simulink model "Modelo_No_lineal_LeyDeControlM"  (R2023b)
settings: Solver=VariableStepAuto  StartTime=0.0  StopTime=10.0  RelTol=1e-3
values from neighbouring files (symbols this model uses):
  alpha_cu = 3.9e-3    (= 0.0039)    [parametros_proyecto2.m]
  g = 9.81    [parametros_proyecto2.m]
  lambda_m = 0.016    [parametros_proyecto2.m]
  Ld = 6.6e-3    (= 0.0066)    [parametros_proyecto2.m]
  Lq = 5.8e-3    (= 0.0058)    [parametros_proyecto2.m]
  r = 120    [parametros_proyecto2.m]
  Rs_ref = 1.02    [parametros_proyecto2.m]
  Rts_amb = 146.7    [parametros_proyecto2.m]
  Ts0 = 25    [parametros_proyecto2.m]
undefined symbols (not defined in the file or in its folder): b_eq, cts, J_eq, k_l, L_d, L_ls, L_q, magnitude, P_p
settings Model: Creator=ignab  LastModifiedBy=MSI

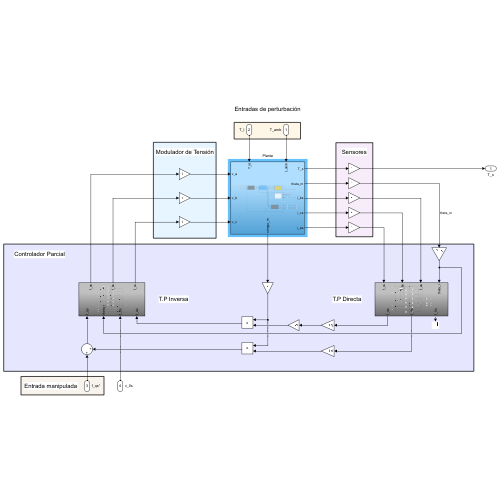
[thumbnail: Simulink's stored preview of the top-level diagram]
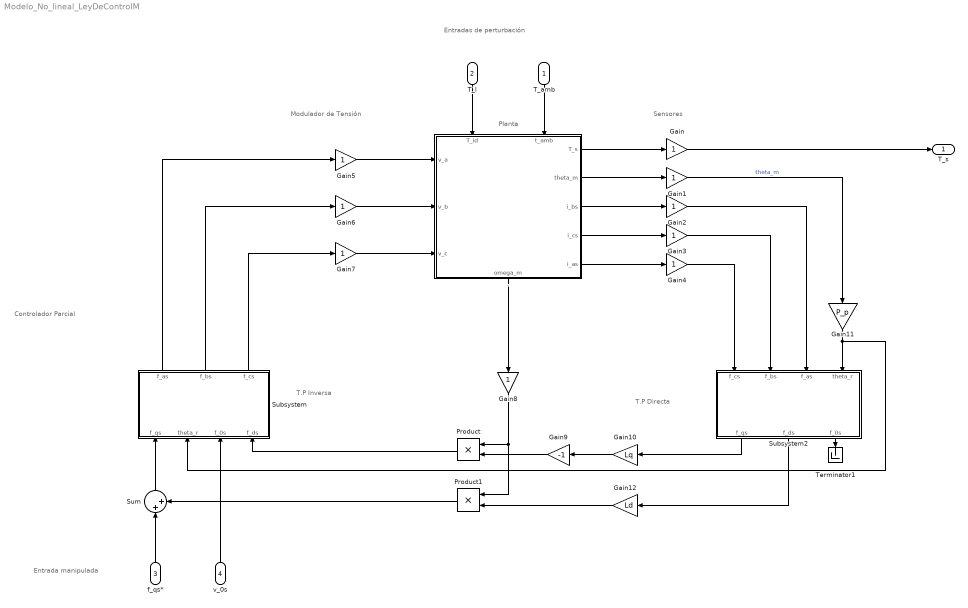
== system Modelo_No_lineal_LeyDeControlM ==
  note: Planta
  note: Modulador de Tensión
  note: Sensores
  note: Entradas de perturbación
  note: Controlador Parcial
  note: T.P Inversa
  note: T.P Directa
  note: Entrada manipulada
  T_amb : Inport
  T_l : Inport  Port=2
  f_qs* : Inport  Port=3
  v_0s : Inport  Port=4
  . : Subsystem
      settings: PortSchema="{\"entries\":[{\"content\":{\"sides\":[{\"content\":{\"connectorIds\":[\"In1\",\"In2\",\"In3\"]},\"type\":\"ConnectorPlacement.EquallySpacedRectSide\",\"uuid\":\"a2221977-a2db-4f9f-a6b6-e4e93ab83132\"},{\"content\":{\"connectorIds\":[\"Out1\",\"Out2\",\"Out3\",\"Out4\",\"Out5\"],\"side\":\"RIGHT\"},\"type\":\"ConnectorPlacement.EquallySpacedRectSide\",\"uuid\":\"4d1b64fb-cd5f-444c-9c55-dd968f667727\"},{\"content\":{\"connectorIds\":[\"In4\",\"In5\"],\"side\":\"TOP\"},\"type\":\"ConnectorPlacement.EquallySpacedRectSide\",\"uuid\":\"feec2d7e-2013-4827-9d2d-5413e6a364ce\"},{\"content\":{\"connectorIds\":[\"Out6\"],\"side\":\"BOTTOM\"},\"type\":\"ConnectorPlacement.EquallySpacedRectSide\",\"uuid\":\"a4e68a75-7272-4a37-88ea-97e0fe693470\"}]},\"type\":\"ConnectorPlacement.EquallySpacedConnector\",\"uuid\":\"3fef7616-1be8-4199-84fe-e5c97ae42ef2\"}],\"packageUris\":[\"http://schema.mathworks.com/mf0/Connector/R2020b\"],\"version\":\"1.0\"}"
  Gain{,1..8} (9 alike) : Gain
  Gain10 : Gain  Gain=Lq
  Gain11 : Gain  Gain=P_p
  Gain12 : Gain  Gain=Ld
  Gain9 : Gain  Gain=-1
  Product : Product
  Product1 : Product
  Subsystem : Subsystem
  Subsystem2 : Subsystem
  Sum : Sum  Inputs=|++
  Terminator1 : Terminator
  T_s : Outport
  wires:
  Subsystem/1(f_as) -> Gain5/1
  Gain5/1 -> ./1(v_a)
  Subsystem/2(f_bs) -> Gain6/1
  Gain6/1 -> ./2(v_b)
  Subsystem/3(f_cs) -> Gain7/1
  Gain7/1 -> ./3(v_c)
  v_0s/1 -> Subsystem/3(f_0s)
  T_l/1 -> ./4(T_id)
  T_amb/1 -> ./5(t_amb)
  ./3(i_bs) -> Gain2/1
  ./4(i_cs) -> Gain3/1
  ./1(T_s) -> Gain/1
  ./2(theta_m) -> Gain1/1
  ./5(i_as) -> Gain4/1
  ./6(omega_m) -> Gain8/1
  Gain/1 -> T_s/1
  Gain1/1 -> Gain11/1  "theta_m"
  Gain11/1 -> Subsystem/2(theta_r), Subsystem2/4(theta_r)
  Gain2/1 -> Subsystem2/3(f_as)
  Gain3/1 -> Subsystem2/2(f_bs)
  Gain4/1 -> Subsystem2/1(f_cs)
  Gain8/1 -> Product1/1, Product/1
  Subsystem2/1(f_qs) -> Gain10/1
  Gain10/1 -> Gain9/1
  Gain9/1 -> Product/2
  Product/1 -> Subsystem/4(f_ds)
  Subsystem2/2(f_ds) -> Gain12/1
  Subsystem2/3(f_0s) -> Terminator1/1
  Gain12/1 -> Product1/2
  f_qs*/1 -> Sum/1
  Sum/1 -> Subsystem/1(f_qs)
  Product1/1 -> Sum/2

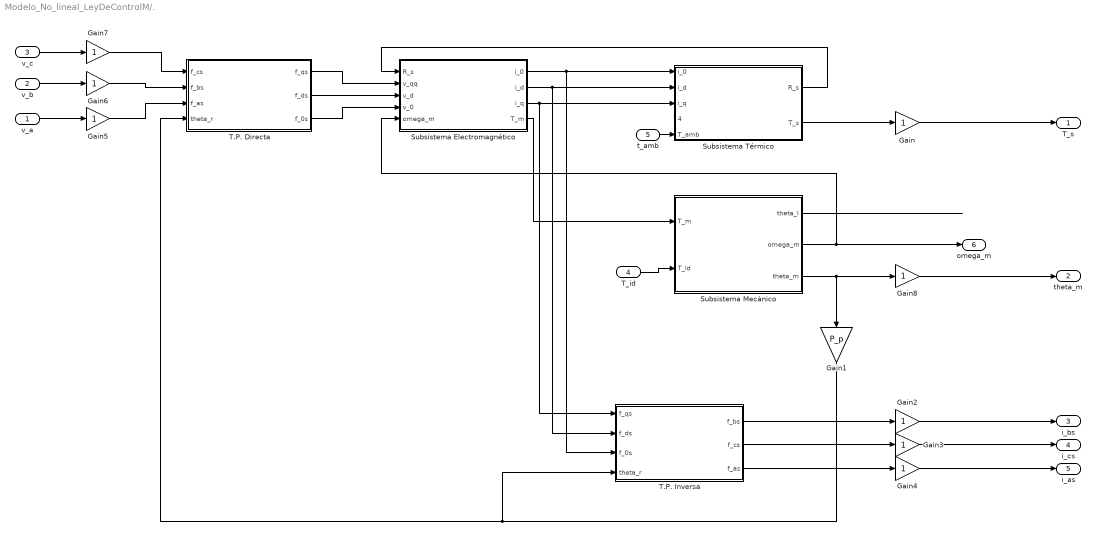
== system Modelo_No_lineal_LeyDeControlM/. ==
  v_a : Inport
  v_b : Inport  Port=2
  v_c : Inport  Port=3
  T_id : Inport  Port=4
  t_amb : Inport  Port=5
  Gain{,2..8} (8 alike) : Gain
  Gain1 : Gain  Gain=P_p
  Subsistema Electromagnético : Subsystem
  Subsistema Mecánico : Subsystem
  Subsistema Térmico : Subsystem
  T.P. Directa : Subsystem
  T.P. Inversa : Subsystem
  T_s : Outport
  theta_m : Outport  Port=2
  i_bs : Outport  Port=3
  i_cs : Outport  Port=4
  i_as : Outport  Port=5
  omega_m : Outport  Port=6
  wires:
  Subsistema Térmico/1(R_s) -> Subsistema Electromagnético/1(R_s)
  T.P. Directa/1(f_qs) -> Subsistema Electromagnético/2(v_qq)
  T.P. Inversa/1(f_bs) -> Gain2/1
  Subsistema Mecánico/2(omega_m) -> Subsistema Electromagnético/5(omega_m), omega_m/1
  Subsistema Electromagnético/1(i_0) -> Subsistema Térmico/1(i_0), T.P. Inversa/3(f_0s)
  Subsistema Mecánico/3(theta_m) -> Gain1/1, Gain8/1
  Gain6/1 -> T.P. Directa/2(f_bs)
  Subsistema Electromagnético/4(T_m) -> Subsistema Mecánico/1(T_m)
  Gain3/1 -> i_cs/1
  Subsistema Mecánico/1(theta_l) -> ?
  Subsistema Electromagnético/2(i_d) -> T.P. Inversa/2(f_ds), Subsistema Térmico/2(i_d)
  Gain2/1 -> i_bs/1
  t_amb/1 -> Subsistema Térmico/5(T_amb)
  v_b/1 -> Gain6/1
  v_c/1 -> Gain7/1
  v_a/1 -> Gain5/1
  Subsistema Térmico/2(T_s) -> Gain/1
  Subsistema Electromagnético/3(i_q) -> T.P. Inversa/1(f_qs), Subsistema Térmico/3(i_q)
  Gain4/1 -> i_as/1
  T.P. Inversa/3(f_as) -> Gain4/1
  T.P. Directa/3(f_0s) -> Subsistema Electromagnético/4(v_0)
  T_id/1 -> Subsistema Mecánico/2(T_ld)
  T.P. Inversa/2(f_cs) -> Gain3/1
  Gain8/1 -> theta_m/1
  Gain7/1 -> T.P. Directa/1(f_cs)
  Gain/1 -> T_s/1
  Gain1/1 -> T.P. Directa/4(theta_r), T.P. Inversa/4(theta_r)
  T.P. Directa/2(f_ds) -> Subsistema Electromagnético/3(v_d)
  Gain5/1 -> T.P. Directa/3(f_as)

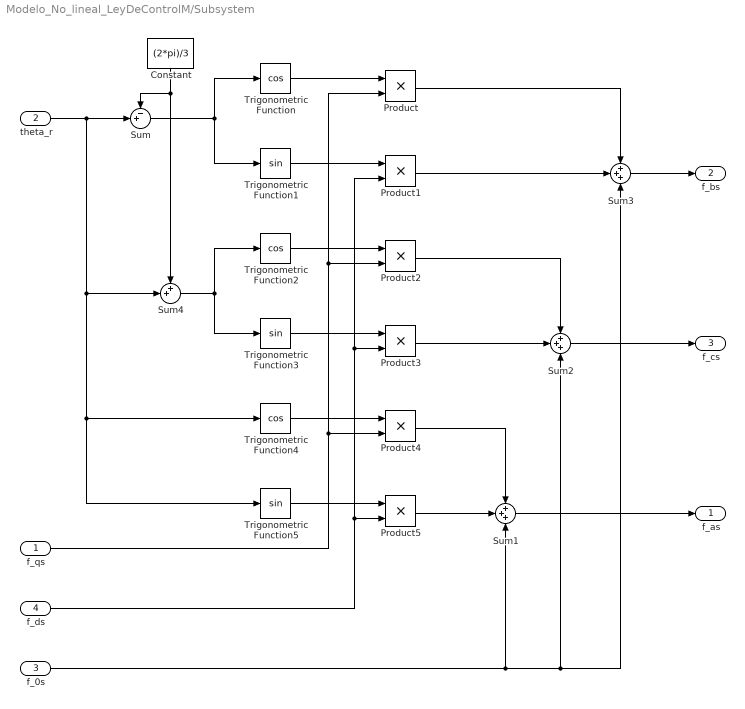
== system Modelo_No_lineal_LeyDeControlM/Subsystem ==
  f_qs : Inport
  theta_r : Inport  Port=2
  f_0s : Inport  Port=3
  f_ds : Inport  Port=4
  Constant : Constant  Value=(2*pi)/3
  Product{,1..5} (6 alike) : Product
  Sum : Sum  Inputs=-+|
  Sum1 : Sum  Inputs=+++
  Sum2 : Sum  Inputs=+++
  Sum3 : Sum  Inputs=+++
  Sum4 : Sum  Inputs=++|
  Trigonometric Function : Trigonometry  Operator=cos
  Trigonometric Function1 : Trigonometry
  Trigonometric Function2 : Trigonometry  Operator=cos
  Trigonometric Function3 : Trigonometry
  Trigonometric Function4 : Trigonometry  Operator=cos
  Trigonometric Function5 : Trigonometry
  f_as : Outport
  f_bs : Outport  Port=2
  f_cs : Outport  Port=3
  wires:
  Sum1/1 -> f_as/1
  Product5/1 -> Sum1/2
  Sum2/1 -> f_cs/1
  Product1/1 -> Sum3/2
  Trigonometric Function5/1 -> Product5/1
  Sum/1 -> Trigonometric Function1/1, Trigonometric Function/1
  Product2/1 -> Sum2/1
  Product4/1 -> Sum1/1
  f_qs/1 -> Product4/2, Product2/2, Product/2
  Product/1 -> Sum3/1
  f_0s/1 -> Sum3/3, Sum2/3, Sum1/3
  Trigonometric Function4/1 -> Product4/1
  Constant/1 -> Sum4/1, Sum/1
  Trigonometric Function2/1 -> Product2/1
  f_ds/1 -> Product5/2, Product3/2, Product1/2
  Trigonometric Function3/1 -> Product3/1
  Trigonometric Function1/1 -> Product1/1
  Sum4/1 -> Trigonometric Function3/1, Trigonometric Function2/1
  Sum3/1 -> f_bs/1
  theta_r/1 -> Sum4/2, Trigonometric Function5/1, Trigonometric Function4/1, Sum/2
  Product3/1 -> Sum2/2
  Trigonometric Function/1 -> Product/1

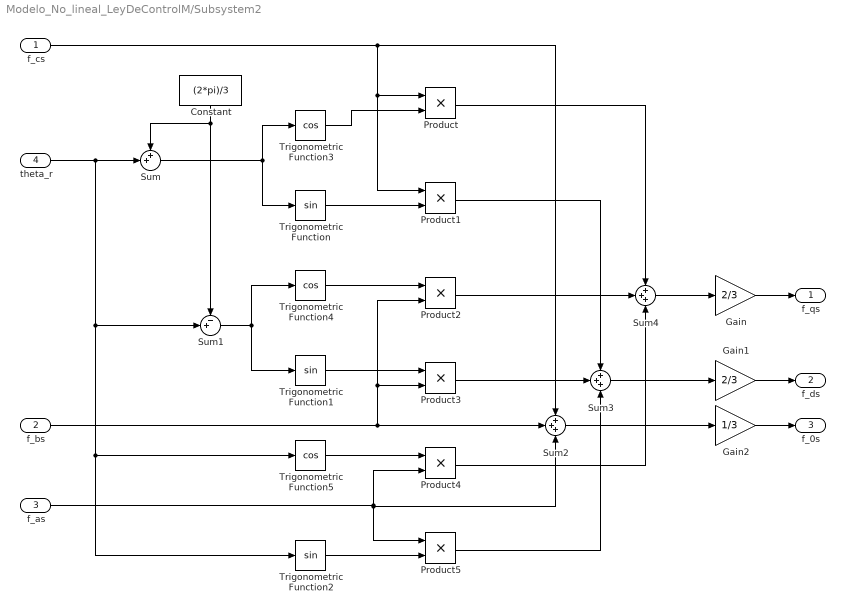
== system Modelo_No_lineal_LeyDeControlM/Subsystem2 ==
  f_cs : Inport
  f_bs : Inport  Port=2
  f_as : Inport  Port=3
  theta_r : Inport  Port=4
  Constant : Constant  Value=(2*pi)/3
  Gain : Gain  Gain=2/3
  Gain1 : Gain  Gain=2/3
  Gain2 : Gain  Gain=1/3
  Product{,1..5} (6 alike) : Product
  Sum : Sum  Inputs=++|
  Sum1 : Sum  Inputs=-+|
  Sum2 : Sum  Inputs=+++
  Sum3 : Sum  Inputs=+++
  Sum4 : Sum  Inputs=+++
  Trigonometric Function : Trigonometry
  Trigonometric Function1 : Trigonometry
  Trigonometric Function2 : Trigonometry
  Trigonometric Function3 : Trigonometry  Operator=cos
  Trigonometric Function4 : Trigonometry  Operator=cos
  Trigonometric Function5 : Trigonometry  Operator=cos
  f_qs : Outport
  f_ds : Outport  Port=2
  f_0s : Outport  Port=3
  wires:
  f_cs/1 -> Product/1, Product1/1, Sum2/1
  Product3/1 -> Sum3/2
  Trigonometric Function5/1 -> Product4/1
  Constant/1 -> Sum/1, Sum1/1
  Sum1/1 -> Trigonometric Function1/1, Trigonometric Function4/1
  Gain2/1 -> f_0s/1
  Gain1/1 -> f_ds/1
  theta_r/1 -> Sum1/2, Trigonometric Function2/1, Trigonometric Function5/1, Sum/2
  Sum4/1 -> Gain/1
  Trigonometric Function1/1 -> Product3/1
  f_bs/1 -> Product2/2, Product3/2, Sum2/2
  Product4/1 -> Sum4/3
  Gain/1 -> f_qs/1
  Product/1 -> Sum4/1
  f_as/1 -> Sum2/3, Product5/1, Product4/2
  Sum2/1 -> Gain2/1
  Product2/1 -> Sum4/2
  Trigonometric Function2/1 -> Product5/2
  Sum3/1 -> Gain1/1
  Trigonometric Function/1 -> Product1/2
  Trigonometric Function3/1 -> Product/2
  Trigonometric Function4/1 -> Product2/1
  Product5/1 -> Sum3/3
  Product1/1 -> Sum3/1
  Sum/1 -> Trigonometric Function3/1, Trigonometric Function/1

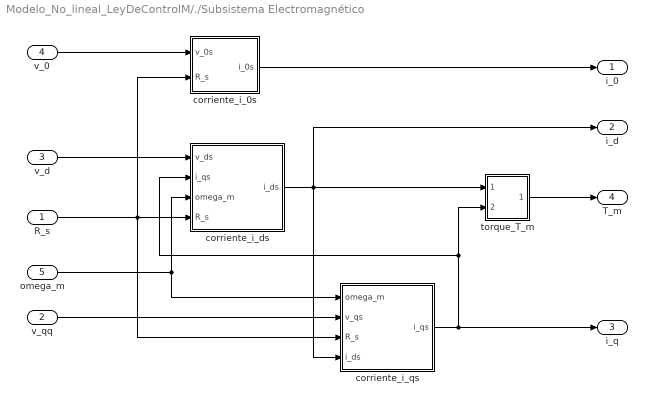
== system Modelo_No_lineal_LeyDeControlM/./Subsistema Electromagnético ==
  R_s : Inport
  v_qq : Inport  Port=2
  v_d : Inport  Port=3
  v_0 : Inport  Port=4
  omega_m : Inport  Port=5
  corriente_i_0s : Subsystem
  corriente_i_ds : Subsystem
  corriente_i_qs : Subsystem
  torque_T_m : Subsystem
  i_0 : Outport
  i_d : Outport  Port=2
  i_q : Outport  Port=3
  T_m : Outport  Port=4
  wires:
  R_s/1 -> corriente_i_qs/3(R_s), corriente_i_ds/4(R_s), corriente_i_0s/2(R_s)
  corriente_i_0s/1(i_0s) -> i_0/1
  corriente_i_qs/1(i_qs) -> i_q/1, torque_T_m/2(i_qs), corriente_i_ds/2(i_qs)
  corriente_i_ds/1(i_ds) -> corriente_i_qs/4(i_ds), torque_T_m/1(i_ds), i_d/1
  v_0/1 -> corriente_i_0s/1(v_0s)
  v_d/1 -> corriente_i_ds/1(v_ds)
  omega_m/1 -> corriente_i_qs/1(omega_m), corriente_i_ds/3(omega_m)
  v_qq/1 -> corriente_i_qs/2(v_qs)
  torque_T_m/1(T_m) -> T_m/1

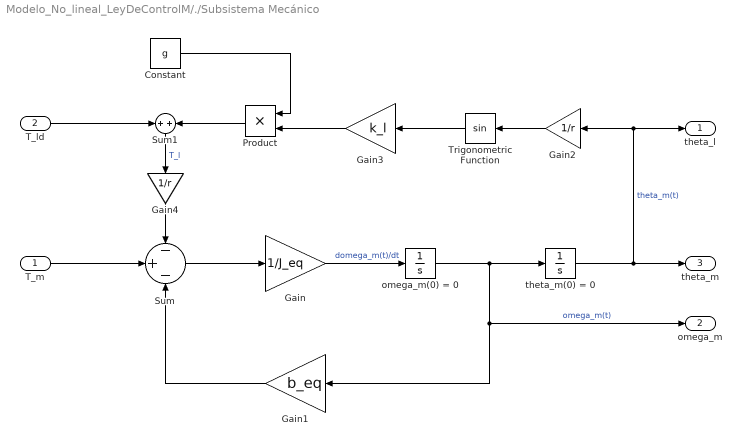
== system Modelo_No_lineal_LeyDeControlM/./Subsistema Mecánico ==
  T_m : Inport
  T_ld : Inport  Port=2
  Constant : Constant  Value=g
  Gain : Gain  Gain=1/J_eq
  Gain1 : Gain  Gain=b_eq
  Gain2 : Gain  Gain=1/r
  Gain3 : Gain  Gain=k_l
  Gain4 : Gain  Gain=1/r
  Product : Product
  Sum : Sum  Inputs=-+-
  Sum1 : Sum
  Trigonometric Function : Trigonometry
  "omega_m(0) = 0\t" : Integrator
  theta_m(0) = 0 : Integrator
  theta_l : Outport
  omega_m : Outport  Port=2
  theta_m : Outport  Port=3
  wires:
  Product/1 -> Sum1/2
  Constant/1 -> Product/1
  T_m/1 -> Sum/2
  Gain3/1 -> Product/2
  T_ld/1 -> Sum1/1
  Gain1/1 -> Sum/3
  Gain4/1 -> Sum/1
  Sum1/1 -> Gain4/1  "T_l"
  theta_m(0) = 0/1 -> theta_l/1, Gain2/1, theta_m/1  "theta_m(t)"
  Trigonometric Function/1 -> Gain3/1
  Sum/1 -> Gain/1
  Gain2/1 -> Trigonometric Function/1
  "omega_m(0) = 0\t"/1 -> theta_m(0) = 0/1, omega_m/1, Gain1/1  "omega_m(t)"
  Gain/1 -> "omega_m(0) = 0\t"/1  "domega_m(t)/dt"

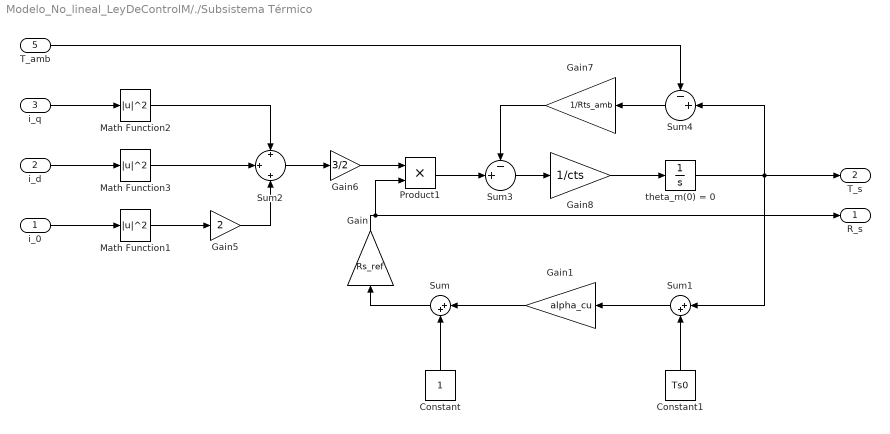
== system Modelo_No_lineal_LeyDeControlM/./Subsistema Térmico ==
  i_0 : Inport
  i_d : Inport  Port=2
  i_q : Inport  Port=3
  T_amb : Inport  Port=5
  Constant : Constant
  Constant1 : Constant  Value=Ts0
  Gain : Gain  Gain=Rs_ref
  Gain1 : Gain  Gain=alpha_cu
  Gain5 : Gain  Gain=2
  Gain6 : Gain  Gain=3/2
  Gain7 : Gain  Gain=1/Rts_amb
  Gain8 : Gain  Gain=1/cts
  Math Function1 : Math  Operator=magnitude^2  OutputSignalType=real
  Math Function2 : Math  Operator=magnitude^2  OutputSignalType=real
  Math Function3 : Math  Operator=magnitude^2  OutputSignalType=real
  Product1 : Product
  Sum : Sum  Inputs=|++
  Sum1 : Sum  Inputs=|++
  Sum2 : Sum  Inputs=+|+|+
  Sum3 : Sum  Inputs=-+|
  Sum4 : Sum  Inputs=-+|
  theta_m(0) = 0 : Integrator
  R_s : Outport
  T_s : Outport  Port=2
  wires:
  i_q/1 -> Math Function2/1
  i_d/1 -> Math Function3/1
  i_0/1 -> Math Function1/1
  Gain1/1 -> Sum/1
  Gain8/1 -> theta_m(0) = 0/1
  Sum3/1 -> Gain8/1
  Constant/1 -> Sum/2
  Product1/1 -> Sum3/2
  Sum/1 -> Gain/1
  T_amb/1 -> Sum4/1
  Math Function1/1 -> Gain5/1
  Sum4/1 -> Gain7/1
  theta_m(0) = 0/1 -> Sum4/2, Sum1/1, T_s/1
  Sum2/1 -> Gain6/1
  Sum1/1 -> Gain1/1
  Gain6/1 -> Product1/1
  Constant1/1 -> Sum1/2
  Gain5/1 -> Sum2/3
  Gain7/1 -> Sum3/1
  Math Function2/1 -> Sum2/1
  Math Function3/1 -> Sum2/2
  Gain/1 -> R_s/1, Product1/2

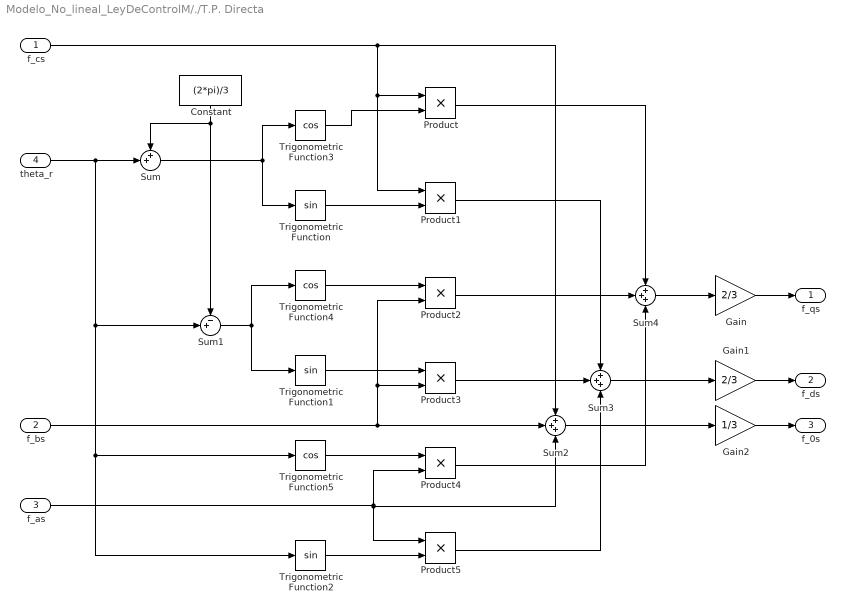
== system Modelo_No_lineal_LeyDeControlM/./T.P. Directa ==
  f_cs : Inport
  f_bs : Inport  Port=2
  f_as : Inport  Port=3
  theta_r : Inport  Port=4
  Constant : Constant  Value=(2*pi)/3
  Gain : Gain  Gain=2/3
  Gain1 : Gain  Gain=2/3
  Gain2 : Gain  Gain=1/3
  Product{,1..5} (6 alike) : Product
  Sum : Sum  Inputs=++|
  Sum1 : Sum  Inputs=-+|
  Sum2 : Sum  Inputs=+++
  Sum3 : Sum  Inputs=+++
  Sum4 : Sum  Inputs=+++
  Trigonometric Function : Trigonometry
  Trigonometric Function1 : Trigonometry
  Trigonometric Function2 : Trigonometry
  Trigonometric Function3 : Trigonometry  Operator=cos
  Trigonometric Function4 : Trigonometry  Operator=cos
  Trigonometric Function5 : Trigonometry  Operator=cos
  f_qs : Outport
  f_ds : Outport  Port=2
  f_0s : Outport  Port=3
  wires:
  Product5/1 -> Sum3/3
  theta_r/1 -> Sum1/2, Trigonometric Function2/1, Trigonometric Function5/1, Sum/2
  f_bs/1 -> Product2/2, Product3/2, Sum2/2
  f_cs/1 -> Product/1, Product1/1, Sum2/1
  Trigonometric Function5/1 -> Product4/1
  Sum1/1 -> Trigonometric Function1/1, Trigonometric Function4/1
  Constant/1 -> Sum/1, Sum1/1
  Sum/1 -> Trigonometric Function3/1, Trigonometric Function/1
  f_as/1 -> Sum2/3, Product5/1, Product4/2
  Gain2/1 -> f_0s/1
  Trigonometric Function2/1 -> Product5/2
  Trigonometric Function1/1 -> Product3/1
  Product/1 -> Sum4/1
  Sum4/1 -> Gain/1
  Trigonometric Function3/1 -> Product/2
  Gain/1 -> f_qs/1
  Gain1/1 -> f_ds/1
  Product2/1 -> Sum4/2
  Product1/1 -> Sum3/1
  Product4/1 -> Sum4/3
  Product3/1 -> Sum3/2
  Sum2/1 -> Gain2/1
  Trigonometric Function4/1 -> Product2/1
  Trigonometric Function/1 -> Product1/2
  Sum3/1 -> Gain1/1

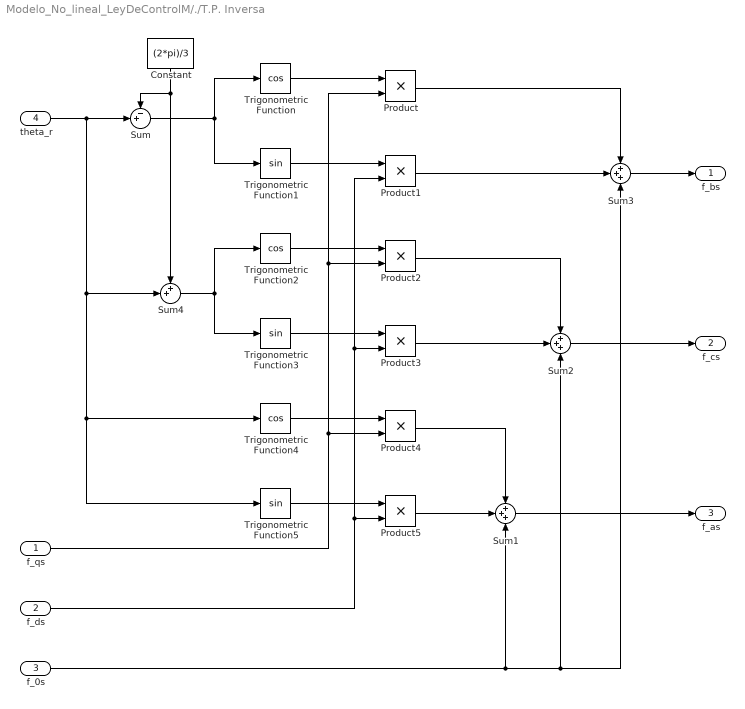
== system Modelo_No_lineal_LeyDeControlM/./T.P. Inversa ==
  f_qs : Inport
  f_ds : Inport  Port=2
  f_0s : Inport  Port=3
  theta_r : Inport  Port=4
  Constant : Constant  Value=(2*pi)/3
  Product{,1..5} (6 alike) : Product
  Sum : Sum  Inputs=-+|
  Sum1 : Sum  Inputs=+++
  Sum2 : Sum  Inputs=+++
  Sum3 : Sum  Inputs=+++
  Sum4 : Sum  Inputs=++|
  Trigonometric Function : Trigonometry  Operator=cos
  Trigonometric Function1 : Trigonometry
  Trigonometric Function2 : Trigonometry  Operator=cos
  Trigonometric Function3 : Trigonometry
  Trigonometric Function4 : Trigonometry  Operator=cos
  Trigonometric Function5 : Trigonometry
  f_bs : Outport
  f_cs : Outport  Port=2
  f_as : Outport  Port=3
  wires:
  theta_r/1 -> Sum4/2, Trigonometric Function5/1, Trigonometric Function4/1, Sum/2
  Trigonometric Function3/1 -> Product3/1
  Product4/1 -> Sum1/1
  Product1/1 -> Sum3/2
  Trigonometric Function2/1 -> Product2/1
  Product2/1 -> Sum2/1
  f_0s/1 -> Sum3/3, Sum2/3, Sum1/3
  f_qs/1 -> Product4/2, Product2/2, Product/2
  Product5/1 -> Sum1/2
  Trigonometric Function1/1 -> Product1/1
  Sum/1 -> Trigonometric Function1/1, Trigonometric Function/1
  Trigonometric Function5/1 -> Product5/1
  Sum4/1 -> Trigonometric Function3/1, Trigonometric Function2/1
  Product/1 -> Sum3/1
  Product3/1 -> Sum2/2
  Trigonometric Function/1 -> Product/1
  Sum2/1 -> f_cs/1
  Sum3/1 -> f_bs/1
  f_ds/1 -> Product5/2, Product3/2, Product1/2
  Trigonometric Function4/1 -> Product4/1
  Sum1/1 -> f_as/1
  Constant/1 -> Sum4/1, Sum/1

== system Modelo_No_lineal_LeyDeControlM/./Subsistema Electromagnético/corriente_i_0s ==
  v_0s : Inport
  R_s : Inport  Port=2
  Gain : Gain  Gain=1/L_ls
  Integrator : Integrator
  Product : Product
  Sum : Sum  Inputs=+-
  i_0s : Outport
  wires:
  Sum/1 -> Gain/1
  Gain/1 -> Integrator/1  "i'_0s"
  Integrator/1 -> i_0s/1, Product/2
  Product/1 -> Sum/2
  v_0s/1 -> Sum/1
  R_s/1 -> Product/1

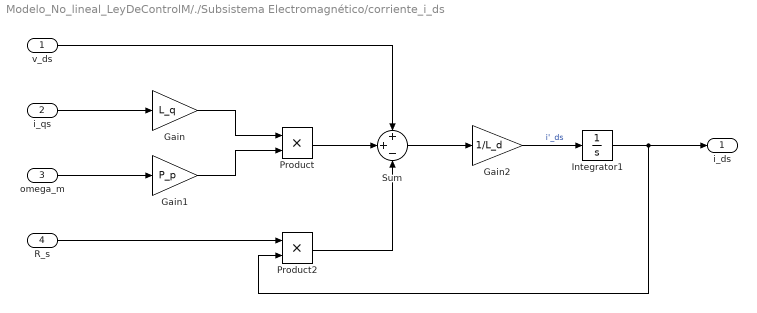
== system Modelo_No_lineal_LeyDeControlM/./Subsistema Electromagnético/corriente_i_ds ==
  v_ds : Inport
  i_qs : Inport  Port=2
  omega_m : Inport  Port=3
  R_s : Inport  Port=4
  Gain : Gain  Gain=L_q
  Gain1 : Gain  Gain=P_p
  Gain2 : Gain  Gain=1/L_d
  Integrator1 : Integrator
  Product : Product
  Product2 : Product
  Sum : Sum  Inputs=++-
  i_ds : Outport
  wires:
  Gain1/1 -> Product/2
  Gain/1 -> Product/1
  i_qs/1 -> Gain/1
  Product/1 -> Sum/2
  Integrator1/1 -> i_ds/1, Product2/2
  v_ds/1 -> Sum/1
  Gain2/1 -> Integrator1/1  "i'_ds"
  R_s/1 -> Product2/1
  Sum/1 -> Gain2/1
  Product2/1 -> Sum/3
  omega_m/1 -> Gain1/1

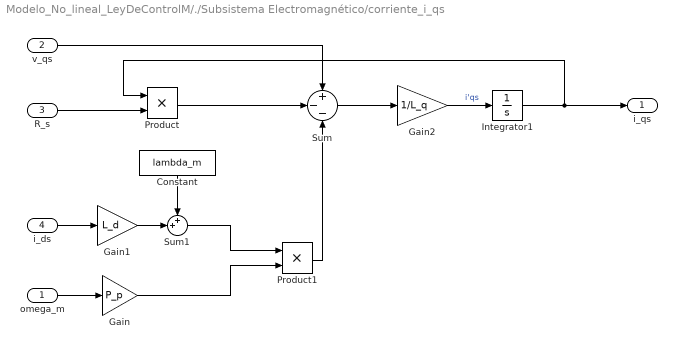
== system Modelo_No_lineal_LeyDeControlM/./Subsistema Electromagnético/corriente_i_qs ==
  omega_m : Inport
  v_qs : Inport  Port=2
  R_s : Inport  Port=3
  i_ds : Inport  Port=4
  Constant : Constant  Value=lambda_m
  Gain : Gain  Gain=P_p
  Gain1 : Gain  Gain=L_d
  Gain2 : Gain  Gain=1/L_q
  Integrator1 : Integrator
  Product : Product
  Product1 : Product
  Sum : Sum  Inputs=+--
  Sum1 : Sum  Inputs=++|
  i_qs : Outport
  wires:
  Gain1/1 -> Sum1/2
  Product/1 -> Sum/2
  R_s/1 -> Product/2
  Sum1/1 -> Product1/1
  v_qs/1 -> Sum/1
  Gain/1 -> Product1/2
  Gain2/1 -> Integrator1/1  "i'qs"
  Constant/1 -> Sum1/1
  i_ds/1 -> Gain1/1
  Sum/1 -> Gain2/1
  omega_m/1 -> Gain/1
  Integrator1/1 -> i_qs/1, Product/1
  Product1/1 -> Sum/3

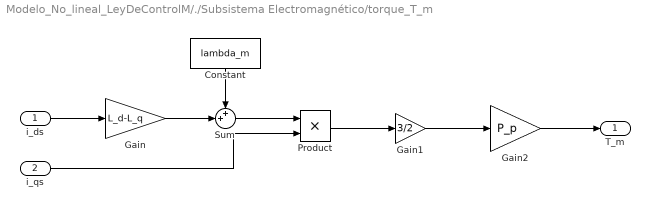
== system Modelo_No_lineal_LeyDeControlM/./Subsistema Electromagnético/torque_T_m ==
  i_ds : Inport
  i_qs : Inport  Port=2
  Constant : Constant  Value=lambda_m
  Gain : Gain  Gain=L_d-L_q
  Gain1 : Gain  Gain=3/2
  Gain2 : Gain  Gain=P_p
  Product : Product
  Sum : Sum  Inputs=++|
  T_m : Outport
  wires:
  Constant/1 -> Sum/1
  Gain/1 -> Sum/2
  i_ds/1 -> Gain/1
  Product/1 -> Gain1/1
  i_qs/1 -> Product/2
  Sum/1 -> Product/1
  Gain1/1 -> Gain2/1
  Gain2/1 -> T_m/1
